simulink model "on_off"  (R2016a)
settings: Solver=FixedStepAuto  StartTime=0.0  StopTime=30  FixedStep=0.01  MaxStep=0.01  RelTol=1e-3
model workspace (MAT data in the model file):
  c = 1
  k = 2
  m = 3
settings Model: Creator=The MathWorks, Inc.  LastModifiedBy=Hamid
settings DataIOCC: LimitDataPoints=on  SaveFormat=Array  SignalLogging=off
settings DebuggingCC: AllowSymbolicDim=off
settings HardwareCC: ProdBitPerPointer=32  ProdLargestAtomicFloat=None  ProdIntDivRoundTo=Undefined  ProdEndianess=Unspecified  ProdWordSize=32  ProdHWDeviceType=32-bit Generic
settings ModelReferenceCC: PropagateSignalLabelsOutOfModel=off
settings ConfigComp: CovModelRefEnable=Off

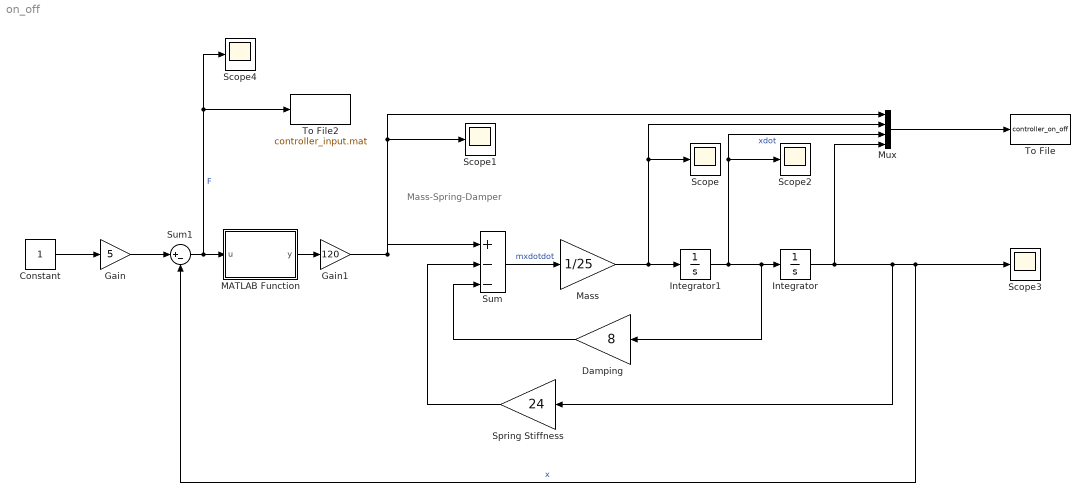
== system on_off ==
  note: Mass-Spring-Damper
  Constant : Constant
  Damping : Gain  Gain=8
  Gain : Gain  Gain=5
  Gain1 : Gain  Gain=120
  Integrator : Integrator
  Integrator1 : Integrator
  MATLAB Function : MATLAB Function  TreatAsAtomicUnit=on
  Mass : Gain  Gain=1/25
  Mux : Mux
  Scope{,1..4} (5 alike) : Scope
  Spring Stiffness : Gain  Gain=24
  Sum : Sum  Inputs=|+--
  Sum1 : Sum  Inputs=|+-
  To File : ToFile  Filename=controller_on_off  MatrixName=controller_on_off  SaveFormat=Timeseries
  To File2 : ToFile  Filename=controller_input.mat  MatrixName=controller_input  SaveFormat=Timeseries
  wires:
  Integrator/1 -> Mux/4, Scope3/1, Sum1/2, Spring Stiffness/1  "x"
  Integrator1/1 -> Scope2/1, Mux/3, Integrator/1, Damping/1  "xdot"
  Damping/1 -> Sum/3
  Spring Stiffness/1 -> Sum/2
  Sum/1 -> Mass/1  "mxdotdot"
  Mass/1 -> Scope/1, Mux/2, Integrator1/1
  Mux/1 -> To File/1
  Constant/1 -> Gain/1
  Gain/1 -> Sum1/1
  Gain1/1 -> Scope1/1, Mux/1, Sum/1
  Sum1/1 -> Scope4/1, To File2/1, MATLAB Function/1(u)  "F"
  MATLAB Function/1(y) -> Gain1/1

== matlab function on_off/MATLAB Function ==
  data: u input; y output
function y = fcn(u)
%#codegen
if u < 0
    y = -1;
else 
    y = 1;
end
